simulink library "OJProbePoint"  (R2019b)
settings: Solver=VariableStepAuto  StartTime=0.0  StopTime=10.0  RelTol=1e-3
settings Model: Creator=kl13806  LastModifiedBy=ra1043664

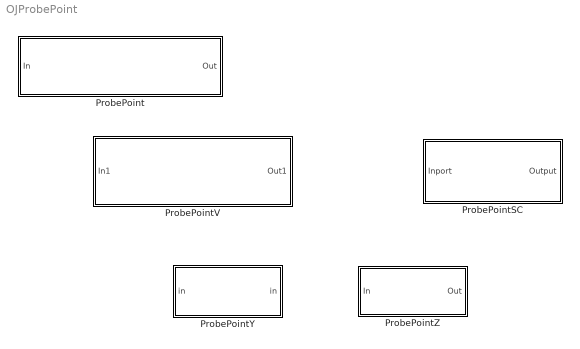
== system OJProbePoint ==
  ProbePoint : Subsystem  Variant=on  mask(ProbePoint){KeyID=0}
      mask prompts: KeyID "Unique Key ID"
      mask help:
      | This block calls the C function "propoint" in generated code assuming this signature:
      |      void probe_point(uint32_t key);
      |
      | Make sure to take some type of action to ensure that the "probe_point" function is at least declared because this block does not.
      |
      | Variants:
      | There are two variants: (1) coder (2) passthro
      | probepoint_coder == true selects the coder variant
      | probepoint_coder == false selects the passthro variant
      mask init:
      | KeyID = uint32(KeyID);
      mask Display: disp('ProbePoint');
  ProbePointSC : Subsystem  mask(Probe Point){probePointEnable=0, probePointID=0}
      mask prompts: probePointEnable "Enable"; probePointID "Unique Key ID"
      mask help:
      | This block calls the C function "probe_point" in generated code assuming this signature:
      |      void probe_point(uint32_t probePointID);
      mask init:
      | probePointID = uint32(probePointID);
      mask Display: disp('OJProbe')
  ProbePointV : Subsystem  Variant=on  mask{Enable=0, ID=0}
      mask prompts: ID "Unique Key ID"
      mask init:
      | probePointID = uint32(ID);
      | %probePointBlk = gcb;
      | %if Enable == true
      | %    set_param(probePointBlk, 'OverrideUsingVariant', 'variant_coder');
      | %else
      | %    set_param(probePointBlk, 'OverrideUsingVariant', 'variant_passthro');
      | %end
  ProbePointY : MATLAB Function  TreatAsAtomicUnit=on  mask(ProbePoint){KeyID=0}
      mask prompts: KeyID "Unique Key ID"
      mask help:
      | This block calls the C function "propoint" in generated code assuming this signature:
      |      void probe_point(uint32_t key);
      |
      | Make sure to take some type of action to ensure that the "probe_point" function is at least declared because this block does not.
      mask init:
      | KeyID = uint32(KeyID);
      settings: RTWSystemCode=Inline
  ProbePointZ : Subsystem  VariantControl=probepoint_coder == false  mask{KeyID=0}
      mask prompts: KeyID "Unique Key ID"
      settings: RTWSystemCode=Inline
      mask Display: disp('ProbePoint');

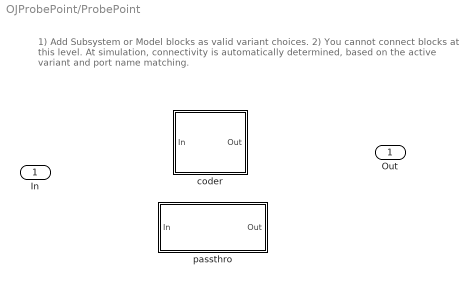
== system OJProbePoint/ProbePoint ==
  note: 1) Add Subsystem or Model blocks as valid variant choices.
      | 2) You cannot connect blocks at this level. At simulation, connectivity is automatically
      | determined, based on the active variant and port name matching.
  In : Inport
  coder : Subsystem  VariantControl=probepoint_coder == true
  passthro : Subsystem  VariantControl=probepoint_coder == false
  Out : Outport

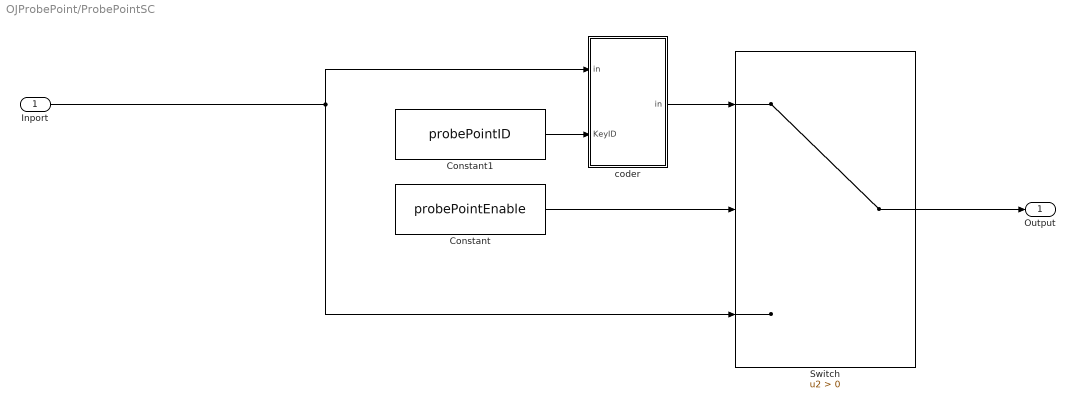
== system OJProbePoint/ProbePointSC ==
  Inport : Inport
  Constant : Constant  Value=probePointEnable  OutDataTypeStr=boolean
  Constant1 : Constant  Value=probePointID  OutDataTypeStr=uint32
  Switch : Switch  Criteria=u2 > Threshold
  coder : MATLAB Function
  Output : Outport
  wires:
  Constant/1 -> Switch/2
  Inport/1 -> coder/1("in "), Switch/3
  Switch/1 -> Output/1
  coder/1(in) -> Switch/1
  Constant1/1 -> coder/2(KeyID)

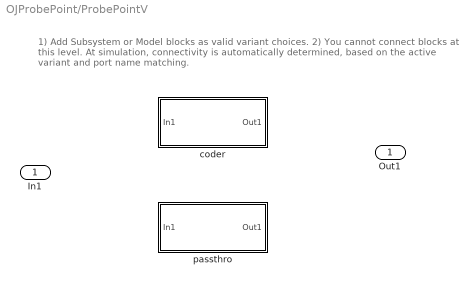
== system OJProbePoint/ProbePointV ==
  note: 1) Add Subsystem or Model blocks as valid variant choices.
      | 2) You cannot connect blocks at this level. At simulation, connectivity is automatically
      | determined, based on the active variant and port name matching.
  In1 : Inport
  coder : Subsystem  VariantControl=probepoint_coder == true
  passthro : Subsystem  VariantControl=probepoint_coder == false
  Out1 : Outport

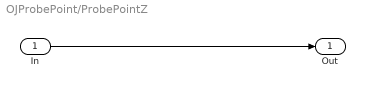
== system OJProbePoint/ProbePointZ ==
  In : Inport
  Out : Outport
  wires:
  In/1 -> Out/1

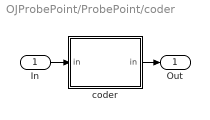
== system OJProbePoint/ProbePoint/coder ==
  In : Inport
  coder : MATLAB Function  TreatAsAtomicUnit=on  VariantControl=probepoint_coder == true
      settings: RTWSystemCode=Inline
  Out : Outport
  wires:
  coder/1(in) -> Out/1
  In/1 -> coder/1("in ")

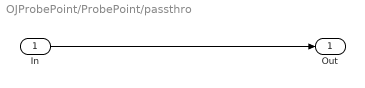
== system OJProbePoint/ProbePoint/passthro ==
  In : Inport
  Out : Outport
  wires:
  In/1 -> Out/1

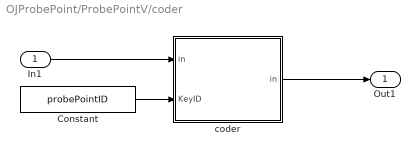
== system OJProbePoint/ProbePointV/coder ==
  In1 : Inport
  Constant : Constant  Value=probePointID  VectorParams1D=off  OutDataTypeStr=uint32
  coder : MATLAB Function
  Out1 : Outport
  wires:
  Constant/1 -> coder/2(KeyID)
  In1/1 -> coder/1("in ")
  coder/1(in) -> Out1/1

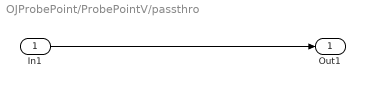
== system OJProbePoint/ProbePointV/passthro ==
  In1 : Inport
  Out1 : Outport
  wires:
  In1/1 -> Out1/1

== matlab function OJProbePoint/ProbePointY ==
  data: in input; in output; KeyID parameter uint32
function in = fcn(in,KeyID)
if (coder.target('Rtw'))
    % Code generation:
     coder.ceval('probe_point',KeyID);
end

== matlab function OJProbePoint/ProbePointSC/coder ==
  data: in input; in output; KeyID input
function in = fcn(in,KeyID)
if (coder.target('Rtw'))
    % Code generation:
     coder.ceval('probe_point',KeyID);
end

== matlab function OJProbePoint/ProbePointV/coder/coder ==
  data: in input; in output; KeyID input
function in = fcn(in,KeyID)
if (coder.target('Rtw'))
    % Code generation:
     coder.ceval('probe_point',KeyID);
end

== matlab function OJProbePoint/ProbePoint/coder/coder ==
  data: in input; in output; KeyID parameter uint32
function in = fcn(in,KeyID)
if (coder.target('Rtw'))
    % Code generation:
     coder.ceval('probe_point',KeyID);
end
